simulink model "Model_pH_and_level_V1"  (Simulink 8.3)
settings: Solver=ode1  SolverMode=SingleTasking  StartTime=0.0  StopTime=Tsim  FixedStep=delta_sim  RelTol=1e-7
values from neighbouring files (symbols this model uses):
  b = 0    [Configuring_pH_and_level_model.m]
  delta_sim = 0.05    [Simulating_pH_and_level_model.m]
  e1 = 50    [Configuring_pH_and_level_model.m]
  e2 = 300    [Configuring_pH_and_level_model.m]
  filter_estimator1 = 1    [Configuring_pH_and_level_model.m]
  filter_estimator2 = 1    [Configuring_pH_and_level_model.m]
  filter_estimator3 = 1    [Configuring_pH_and_level_model.m]
  filter_estimator4 = 1    [Configuring_pH_and_level_model.m]
  filter_estimator5 = 1    [Configuring_pH_and_level_model.m]
  filter_estimator6 = 1    [Configuring_pH_and_level_model.m]
  filtro_Kp = fir1(5,1/50)    [Configuring_pH_and_level_model.m]
  filtro_med_F_TAPI = 1    [Configuring_pH_and_level_model.m]
  filtro_med_F_TASI = 1    [Configuring_pH_and_level_model.m]
  filtro_med_pH = 1    [Configuring_pH_and_level_model.m]
  filtro_Ti = fir1(5,1/50)    [Configuring_pH_and_level_model.m]
  h_max_TR_m = 0.5    [Configuring_pH_and_level_model.m]
  h_nom = 75    [Configuring_pH_and_level_model.m]
  I_l = 271.52    [Configuring_pH_and_level_model.m]
  K_meter_flow = 3600    [Configuring_pH_and_level_model.m]
  K_meter_level = 1    [Configuring_pH_and_level_model.m]
  K_meter_pH = 1    [Configuring_pH_and_level_model.m]
  Kc = 3.5    [Configuring_pH_and_level_model.m]
  Kn = 100/14    (= 7.14285714286)    [Configuring_pH_and_level_model.m]
  Kv = 11e-2    (= 0.11)    [Configuring_pH_and_level_model.m]
  mv0 = 50    [Configuring_pH_and_level_model.m]
  N = 1/500    (= 0.002)    [Configuring_pH_and_level_model.m]
  P_l = 11.65    [Configuring_pH_and_level_model.m]
  pH_nom = 7    [Configuring_pH_and_level_model.m]
  pka1_CH3COOH = interp1(Temp,pK_CH3COOH,T)    [Configuring_pH_and_level_model.m]
  pka1_H2CO3 = interp1(Temp,pK_H2CO3,T)    [Configuring_pH_and_level_model.m]
  pka1_H3PO4 = interp1(Temp,pK_H3PO4,T)    [Configuring_pH_and_level_model.m]
  pka1_NH4 = interp1(Temp,pK_NH4,T)    [Configuring_pH_and_level_model.m]
  pka2_H2CO3 = interp1(Temp,pK_HCO3,T)    [Configuring_pH_and_level_model.m]
  pka2_H3PO4 = interp1(Temp,pK_H2PO4,T)    [Configuring_pH_and_level_model.m]
  pka3_H3PO4 = interp1(Temp,pK_HPO4,T)    [Configuring_pH_and_level_model.m]
  pKw = interp1(Temp,pK_H2O,T)    [Configuring_pH_and_level_model.m]
  Q_ap_nom = 49/3600    (= 0.0136111111111)    [Configuring_pH_and_level_model.m]
  Qb_nom = c_HCl/c_NaOH*Q_ap_nom    (= 0.00412773748633)    [Configuring_pH_and_level_model.m]
  seed_noise_level = 12345    [Configuring_pH_and_level_model.m]
  seed_noise_pH = 67890    [Configuring_pH_and_level_model.m]
  seed_noise_Q_ap = 357    [Configuring_pH_and_level_model.m]
  seed_noise_Q_as = 349    [Configuring_pH_and_level_model.m]
  T_noise_level = 2    [Configuring_pH_and_level_model.m]
  T_noise_pH = 3    [Configuring_pH_and_level_model.m]
  T_PWM = 10    [Configuring_pH_and_level_model.m]
  tau_meter_flow = 1.4    [Configuring_pH_and_level_model.m]
  tau_meter_level = 16    [Configuring_pH_and_level_model.m]
  tau_meter_pH = 5    [Configuring_pH_and_level_model.m]
  Td = 120    [Configuring_pH_and_level_model.m]
  td_meter_flow = 3.5    [Configuring_pH_and_level_model.m]
  td_meter_level = 6    [Configuring_pH_and_level_model.m]
  td_meter_pH = 3.5    [Configuring_pH_and_level_model.m]
  Ti = 150    [Configuring_pH_and_level_model.m]
  Tmix = 1.34    [Configuring_pH_and_level_model.m]
  Ts = 0.5    [Simulating_pH_and_level_model.m]
  Ts_F_TAPI = 1    [Configuring_pH_and_level_model.m]
  Ts_F_TASI = 1    [Configuring_pH_and_level_model.m]
  Ts_Kp = 5    [Configuring_pH_and_level_model.m]
  Ts_pH_m = 1    [Configuring_pH_and_level_model.m]
  Ts_Ti = 5    [Configuring_pH_and_level_model.m]
  Ts_w1 = 1    [Configuring_pH_and_level_model.m]
  Ts_w2 = 1    [Configuring_pH_and_level_model.m]
  Ts_w3 = 1    [Configuring_pH_and_level_model.m]
  Ts_w4 = 1    [Configuring_pH_and_level_model.m]
  Ts_w5 = 1    [Configuring_pH_and_level_model.m]
  Ts_w6 = 25    [Configuring_pH_and_level_model.m]
  V0_CSTR = V_max_CSTR*h_nom/h_max_TR    (= 46.3491936722)    [Configuring_pH_and_level_model.m]
  V_max_CSTR = A_util_TR*h_max_TR_m*1000    (= 61.7989248962)    [Configuring_pH_and_level_model.m]
  var_noise_level = 1.1e-3    (= 0.0011)    [Configuring_pH_and_level_model.m]
  var_noise_pH = 6.25e-5    (= 6.25e-05)    [Configuring_pH_and_level_model.m]
  var_noise_Q_ap = 1.56e-2    (= 0.0156)    [Configuring_pH_and_level_model.m]
  var_noise_Q_as = 1.56e-2    (= 0.0156)    [Configuring_pH_and_level_model.m]
  Vm = 0.836    [Configuring_pH_and_level_model.m]
  w1_ff_tap = 0.0056    [Configuring_pH_and_level_model.m]
  w1_ff_tas = 0    [Configuring_pH_and_level_model.m]
  w1_ff_tbb = -0.0185    [Configuring_pH_and_level_model.m]
  w2_ff_tap = 0.5e-4    (= 5e-05)    [Configuring_pH_and_level_model.m]
  w2_ff_tbb = 0.5e-4    (= 5e-05)    [Configuring_pH_and_level_model.m]
  w3_ff_tap = 3e-4    (= 0.0003)    [Configuring_pH_and_level_model.m]
  w3_ff_tas = 3e-4    (= 0.0003)    [Configuring_pH_and_level_model.m]
  w3_ff_tbb = 3e-4    (= 0.0003)    [Configuring_pH_and_level_model.m]
  w4_ff_tap = 2e-4    (= 0.0002)    [Configuring_pH_and_level_model.m]
  w4_ff_tas = 2e-4    (= 0.0002)    [Configuring_pH_and_level_model.m]
  w4_ff_tbb = 2e-4    (= 0.0002)    [Configuring_pH_and_level_model.m]
  w_ap1 = c_HCl    (= 0.0055861204494)    [Configuring_pH_and_level_model.m]
  w_ap2 = c_CH3COOH_r    (= 0.0001)    [Configuring_pH_and_level_model.m]
  w_ap3 = c_H2CO3_r    (= 0.0009)    [Configuring_pH_and_level_model.m]
  w_ap4 = c_NH4    (= 0.0002)    [Configuring_pH_and_level_model.m]
  w_ap5 = c_H3PO4    (= 1e-05)    [Configuring_pH_and_level_model.m]
  w_as1 = 0    [Configuring_pH_and_level_model.m]
  w_as2 = c_CH3COOH    (= 0.00676612574825)    [Configuring_pH_and_level_model.m]
  w_as3 = c_H2CO3_r    (= 0.0009)    [Configuring_pH_and_level_model.m]
  w_as4 = c_NH4    (= 0.0002)    [Configuring_pH_and_level_model.m]
  w_as5 = c_H3PO4    (= 1e-05)    [Configuring_pH_and_level_model.m]
  w_b1 = -c_NaOH    (= -0.0184200924523)    [Configuring_pH_and_level_model.m]
  w_b2 = c_CH3COOH_r    (= 0.0001)    [Configuring_pH_and_level_model.m]
  w_b3 = c_H2CO3    (= 0.0005)    [Configuring_pH_and_level_model.m]
  w_b4 = c_NH4    (= 0.0002)    [Configuring_pH_and_level_model.m]
  w_b5 = c_H3PO4    (= 1e-05)    [Configuring_pH_and_level_model.m]
  w_fb_tap = [w1_ff_tap w2_ff_tap w3_ff_tap w4_ff_tap]    [Configuring_pH_and_level_model.m]
  w_fb_tas = [w1_ff_tas 0 w3_ff_tas w4_ff_tas]    [Configuring_pH_and_level_model.m]
  w_r1_0 = [w1_r1_0; c_CH3COOH_r; c_H2CO3_r; c_NH4; c_H3PO4]    [Configuring_pH_and_level_model.m]
  x_MV_pump = [0 10 20 40 50 60 80 100]    [Configuring_pH_and_level_model.m]
  y_Q_pump = Q_l_h/3600    [Configuring_pH_and_level_model.m]
libraries: simulink x6, simulink_extras x4
(part 1 of 2)
settings Model: Creator=BrIdent  LastModifiedBy=Fellipe
settings DataIOCC: Decimation=Decim  LimitDataPoints=off  SaveOutput=off  SignalLogging=off  TimeSaveName=t
settings OptimizationCC: ExpressionDepthLimit=2147483647
settings DebuggingCC: AlgebraicLoopMsg=none  ArtificialAlgebraicLoopMsg=none  SaveWithDisabledLinksMsg=none  SaveWithParameterizedLinksMsg=none  CheckSSInitialOutputMsg=off  MaxConsecutiveZCsMsg=none  SolverPrmCheckMsg=none  InheritedTsInSrcMsg=none  DiscreteInheritContinuousMsg=none  MultiTaskCondExecSysMsg=none  MultiTaskRateTransMsg=warning  TasksWithSamePriorityMsg=none  SigSpecEnsureSampleTimeMsg=none  Int32ToFloatConvMsg=none  ParameterDowncastMsg=none  ParameterOverflowMsg=none  InvalidFcnCallConnMsg=none  FcnCallInpInsideContextMsg=UseLocalSettings  UnconnectedInputMsg=none  UnconnectedOutputMsg=none  UnconnectedLineMsg=none  BusObjectLabelMismatch=none  RootOutportRequireBusObject=none  UnknownTsInhSupMsg=none  ModelReferenceDataLoggingMessage=none  ModelReferenceExtraNoncontSigs=none  StateNameClashWarn=none
settings ConfigurationSet: Description=SimMechanics 2G

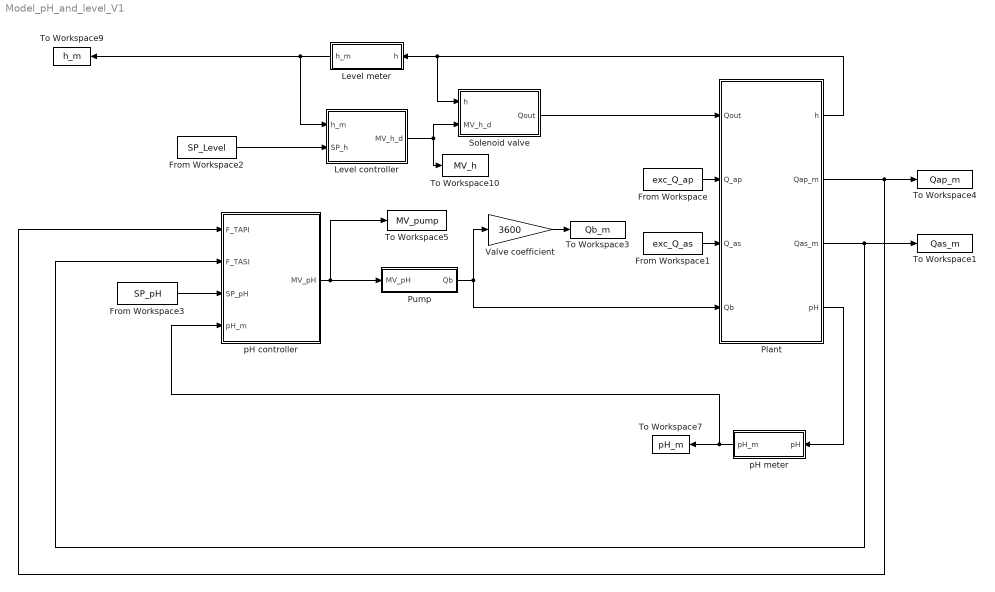
== system Model_pH_and_level_V1 ==
  From Workspace : FromWorkspace  VariableName=exc_Q_ap  SampleTime=1  Interpolate=off  OutputAfterFinalValue=Holding final value
  From Workspace1 : FromWorkspace  VariableName=exc_Q_as  SampleTime=1  Interpolate=off  OutputAfterFinalValue=Holding final value
  From Workspace2 : FromWorkspace  VariableName=SP_Level  SampleTime=1  Interpolate=off  OutputAfterFinalValue=Holding final value
  From Workspace3 : FromWorkspace  VariableName=SP_pH  SampleTime=1  Interpolate=off  OutputAfterFinalValue=Holding final value
  Level controller : Subsystem
  Level meter : Subsystem
  Plant : Subsystem
  Pump : Subsystem
  Solenoid valve : Subsystem
  To Workspace1 : ToWorkspace  VariableName=Qas_m  SampleTime=-1
      settings: Decimation=Ts/delta_sim
  To Workspace10 : ToWorkspace  VariableName=MV_h  SampleTime=-1
      settings: Decimation=Ts/delta_sim
  To Workspace3 : ToWorkspace  VariableName=Qb_m  SampleTime=-1
      settings: Decimation=Ts/delta_sim
  To Workspace4 : ToWorkspace  VariableName=Qap_m  SampleTime=-1
      settings: Decimation=Ts/delta_sim
  To Workspace5 : ToWorkspace  VariableName=MV_pump  SampleTime=-1
      settings: Decimation=Ts/delta_sim
  To Workspace7 : ToWorkspace  VariableName=pH_m  SampleTime=-1
      settings: Decimation=Ts/delta_sim
  To Workspace9 : ToWorkspace  VariableName=h_m  SampleTime=-1
      settings: Decimation=Ts/delta_sim
  Valve coefficient : Gain  Gain=3600
  pH controller : Subsystem  Description=Controlador
  pH meter : Subsystem
  wires:
  pH controller/1(MV_pH) -> To Workspace5/1, Pump/1(MV_pH)
  Plant/4(pH) -> pH meter/1(pH)
  Plant/1(h) -> Level meter/1(h), Solenoid valve/1(h)
  Pump/1(Qb) -> Valve coefficient/1, Plant/4(Qb)
  Plant/2(Qap_m) -> To Workspace4/1, pH controller/1(F_TAPI)
  From Workspace2/1 -> Level controller/2(SP_h)
  From Workspace3/1 -> pH controller/3(SP_pH)
  Level meter/1(h_m) -> Level controller/1(h_m), To Workspace9/1
  Solenoid valve/1(Qout) -> Plant/1(Qout)
  Level controller/1(MV_h_d) -> Solenoid valve/2(MV_h_d), To Workspace10/1
  From Workspace1/1 -> Plant/3(Q_as)
  Plant/3(Qas_m) -> To Workspace1/1, pH controller/2(F_TASI)
  From Workspace/1 -> Plant/2(Q_ap)
  Valve coefficient/1 -> To Workspace3/1
  pH meter/1(pH_m) -> pH controller/4(pH_m), To Workspace7/1

== system Model_pH_and_level_V1/Level controller ==
  h_m : Inport
  SP_h : Inport  Port=2
  PI Controller : simulink/Continuous/PID Controller  Controller=PI  TimeDomain=Discrete-time  SampleTime=Ts  IntegratorMethod=Trapezoidal  FilterMethod=Forward Euler  Form=Ideal  P=P_l  I=I_l  D=0  N=100  InitialConditionSource=internal  InitialConditionForIntegrator=0  InitialConditionForFilter=0  ExternalReset=none  LimitOutput=on  UpperSaturationLimit=100  LowerSaturationLimit=0  LinearizeAsGain=off  AntiWindupMode=back-calculation  Kb=1  TrackingMode=off  Kt=1  PParamMin=[]  PParamMax=[]  IParamMin=[]  IParamMax=[]  DParamMin=[]  DParamMax=[]  NParamMin=[]  NParamMax=[]  KbParamMin=[]  KbParamMax=[]  KtParamMin=[]  KtParamMax=[]  POutMin=[]  POutMax=[]  IOutMin=[]  IOutMax=[]  DOutMin=[]  DOutMax=[]  NOutMin=[]  NOutMax=[]  KbOutMin=[]  KbOutMax=[]  KtOutMin=[]  KtOutMax=[]  IntegratorOutMin=[]  IntegratorOutMax=[]  FilterOutMin=[]  FilterOutMax=[]  SumOutMin=[]  SumOutMax=[]  SumI1OutMin=[]  SumI1OutMax=[]  SumI2OutMin=[]  SumI2OutMax=[]  SumI3OutMin=[]  SumI3OutMax=[]  SumDOutMin=[]  SumDOutMax=[]  SaturationOutMin=[]  SaturationOutMax=[]  IntegratorContinuousStateAttributes=''  IntegratorStateMustResolveToSignalObject=off  IntegratorRTWStateStorageClass=Auto  FilterContinuousStateAttributes=''  FilterStateMustResolveToSignalObject=off  FilterRTWStateStorageClass=Auto
  PWM : Subsystem
  Sum : Sum  Inputs=-+
  MV_h_d : Outport
  wires:
  PI Controller/1 -> PWM/1(MV_h)
  PWM/1(MV_h_d) -> MV_h_d/1
  Sum/1 -> PI Controller/1  "e_h"
  h_m/1 -> Sum/2
  SP_h/1 -> Sum/1

== system Model_pH_and_level_V1/Level meter ==
  h : Inport
  1-D Lookup Table : Lookup_n-D  NumberOfTableDimensions=1  BreakpointsForDimension1=[53.78 62.05 70.32 83.51]  Table=[1.4 1.4 2.21 2.36]  ExtrapMethod=Clip  UseLastTableValue=on  InternalRulePriority=Speed  RndMeth=Simplest  InputSameDT=on
  Add : Sum
  Add1 : Sum
  Close : Constant  Value=0
  From Workspace : FromWorkspace  VariableName=mz81  Interpolate=off  OutputAfterFinalValue=Holding final value
  Level meter : simulink_extras/Additional Linear/Transfer Fcn (with initial outputs)  N=[K_meter_level]  D=[tau_meter_level 1]  Y0=h_nom  U0=h_nom
  Random Number : RandomNumber  Variance=var_noise_level  Seed=seed_noise_level  SampleTime=T_noise_level
  Switch : Switch  Criteria=u2 ~= 0
  Transport Delay : TransportDelay  DelayTime=td_meter_level  InitialOutput=h_nom
  h_m : Outport
  wires:
  h/1 -> 1-D Lookup Table/1, Level meter/1
  Level meter/1 -> Transport Delay/1
  Random Number/1 -> Add/2
  Transport Delay/1 -> Add/1
  Add/1 -> Add1/1
  Add1/1 -> h_m/1
  Close/1 -> Switch/3
  1-D Lookup Table/1 -> Switch/1
  From Workspace/1 -> Switch/2
  Switch/1 -> Add1/2

== system Model_pH_and_level_V1/Plant ==
  Qout : Inport
  Q_ap : Inport  Port=2
  Q_as : Inport  Port=3
  Qb : Inport  Port=4
  Flow meter Qap : Subsystem
  Flow meter Qas : Subsystem
  Plant : Subsystem
  h : Outport
  Qap_m : Outport  Port=2
  Qas_m : Outport  Port=3
  pH : Outport  Port=4
  wires:
  Plant/2(pH) -> pH/1
  Q_ap/1 -> Flow meter Qap/1(Qa), Plant/1(Q_ap)
  Qb/1 -> Plant/3(Qb)
  Flow meter Qap/1(Qap_m) -> Qap_m/1
  Q_as/1 -> Plant/2(Q_as), Flow meter Qas/1(Qa)
  Flow meter Qas/1(Qas_m) -> Qas_m/1
  Plant/1(h) -> h/1
  Qout/1 -> Plant/4(Qout)

== system Model_pH_and_level_V1/Pump ==
  MV_pH : Inport
  1-D Lookup Table : Lookup_n-D  NumberOfTableDimensions=1  BreakpointsForDimension1=x_MV_pump  Table=y_Q_pump  ExtrapMethod=Clip  RndMeth=Simplest  InputSameDT=on
  Qb : Outport
  wires:
  MV_pH/1 -> 1-D Lookup Table/1
  1-D Lookup Table/1 -> Qb/1

== system Model_pH_and_level_V1/Solenoid valve ==
  h : Inport
  MV_h_d : Inport  Port=2
  Conversion of level in % to meter : Gain  Gain=h_max_TR_m/100
  Product : Product  RndMeth=Zero
  Sqrt : Sqrt  SaturateOnIntegerOverflow=on
  Valve coefficient : Gain  Gain=Kv
  Qout : Outport
  wires:
  h/1 -> Conversion of level in % to meter/1
  Valve coefficient/1 -> Product/1
  MV_h_d/1 -> Valve coefficient/1
  Conversion of level in % to meter/1 -> Sqrt/1
  Sqrt/1 -> Product/2
  Product/1 -> Qout/1

== system Model_pH_and_level_V1/pH controller ==
  F_TAPI : Inport  Description=Qref
  F_TASI : Inport  Description=Qref  Port=2
  SP_pH : Inport  Description=Qref  Port=3
  pH_m : Inport  Description=Qref  Port=4
  Demux : Demux  Outputs=3
  Filter : Subsystem
  Mux : Mux  Inputs=3
  PID 2DOF + FF : Subsystem  Description=Controlador
  controller : Subsystem  Description=Controlador
  invariants estimator : Subsystem  Description=Controlador
  MV_pH : Outport
  wires:
  SP_pH/1 -> PID 2DOF + FF/1(SP_pH), controller/1(SP_pH)
  invariants estimator/1(w) -> controller/2(w)
  controller/1(MV_pH) -> MV_pH/1, invariants estimator/1(VM)
  F_TAPI/1 -> PID 2DOF + FF/3(Qap), invariants estimator/2(F_TAPI), Mux/1
  F_TASI/1 -> PID 2DOF + FF/4(Qas), invariants estimator/3(F_TASI), Mux/2
  pH_m/1 -> PID 2DOF + FF/2(pH_m), invariants estimator/4(pH_m), Mux/3
  Mux/1 -> Filter/1(U)
  Filter/1(Y) -> Demux/1
  Demux/1 -> controller/3(F_TAPI)
  Demux/2 -> controller/4(F_TASI)
  Demux/3 -> controller/5(pH_m)

== system Model_pH_and_level_V1/pH meter ==
  pH : Inport
  Add : Sum
  Random Number : RandomNumber  Variance=var_noise_pH  Seed=seed_noise_pH  SampleTime=T_noise_pH
  Transport Delay : TransportDelay  DelayTime=td_meter_pH  InitialOutput=pH_nom
  pH meter : simulink_extras/Additional Linear/Transfer Fcn (with initial outputs)  N=[K_meter_pH]  D=[tau_meter_pH 1]  Y0=pH_nom  U0=pH_nom
  pH_m : Outport
  wires:
  Transport Delay/1 -> Add/1
  Random Number/1 -> Add/2
  pH meter/1 -> Transport Delay/1
  pH/1 -> pH meter/1
  Add/1 -> pH_m/1

== system Model_pH_and_level_V1/Level controller/PWM ==
  MV_h : Inport
  Add1 : Sum  Inputs=++-
  Close : Constant  Value=0
  Compare to Zero : simulink/Logic and Bit Operations/Compare To Zero  relop=<=  OutDataTypeStr=boolean
  Constant : Constant  Value=50
  Open : Constant
  Sawtooth : SignalGenerator  WaveForm=sawtooth  Amplitude=50  Frequency=1/T_PWM
  Switch : Switch  Criteria=u2 > Threshold
  MV_h_d : Outport
  wires:
  Close/1 -> Switch/3
  Open/1 -> Switch/1
  Switch/1 -> MV_h_d/1
  Compare to Zero/1 -> Switch/2
  Constant/1 -> Add1/2
  MV_h/1 -> Add1/3
  Sawtooth/1 -> Add1/1
  Add1/1 -> Compare to Zero/1

== system Model_pH_and_level_V1/Plant/Flow meter Qap ==
  Qa : Inport
  Add : Sum
  Constant : Constant  Value=0
  Flow meter : simulink_extras/Additional Linear/Transfer Fcn (with initial outputs)  N=[K_meter_flow]  D=[tau_meter_flow 1]  Y0=0  U0=0
  Random Number : RandomNumber  Variance=var_noise_Q_ap  Seed=seed_noise_Q_ap  SampleTime=delta_sim
  Switch : Switch  Criteria=u2 > Threshold  Threshold=5/3600
  Transport Delay : TransportDelay  DelayTime=td_meter_flow
  Qap_m : Outport
  wires:
  Random Number/1 -> Add/2
  Qa/1 -> Switch/2, Flow meter/1
  Flow meter/1 -> Transport Delay/1
  Transport Delay/1 -> Add/1
  Add/1 -> Switch/1
  Constant/1 -> Switch/3
  Switch/1 -> Qap_m/1

== system Model_pH_and_level_V1/Plant/Flow meter Qas ==
  Qa : Inport
  Add : Sum
  Constant : Constant  Value=0
  Flow meter : simulink_extras/Additional Linear/Transfer Fcn (with initial outputs)  N=[K_meter_flow]  D=[tau_meter_flow 1]  Y0=0  U0=0
  Random Number : RandomNumber  Variance=var_noise_Q_as  Seed=seed_noise_Q_as  SampleTime=delta_sim
  Switch : Switch  Criteria=u2 > Threshold  Threshold=5/3600
  Transport Delay : TransportDelay  DelayTime=td_meter_flow
  Qas_m : Outport
  wires:
  Qa/1 -> Switch/2, Flow meter/1
  Random Number/1 -> Add/2
  Flow meter/1 -> Transport Delay/1
  Transport Delay/1 -> Add/1
  Constant/1 -> Switch/3
  Add/1 -> Switch/1
  Switch/1 -> Qas_m/1

== system Model_pH_and_level_V1/Plant/Plant ==
  Q_ap : Inport
  Q_as : Inport  Port=2
  Qb : Inport  Port=3
  Qout : Inport  Port=4
  Level model : Subsystem
  Simplified pH model : Subsystem  Description=Controlador
  pH model by reaction invariants : Subsystem
  h : Outport
  pH : Outport  Port=2
  wires:
  Level model/1(h) -> h/1
  pH model by reaction invariants/1(pH) -> pH/1
  Level model/2(V) -> pH model by reaction invariants/5(V)
  Q_ap/1 -> Simplified pH model/3(F_TASI), Level model/1(Q_ap), pH model by reaction invariants/1(Q_ap)
  Q_as/1 -> Simplified pH model/2(F_TAPI), Level model/2(Q_as), pH model by reaction invariants/2(Q_as)
  Qb/1 -> Simplified pH model/1(F_TBB), Level model/3(Qb), pH model by reaction invariants/3(Qb)
  Qout/1 -> Level model/4(Qout), pH model by reaction invariants/4(Qout)

== system Model_pH_and_level_V1/pH controller/Filter ==
  U : Inport
  Demux : Demux  Outputs=3
  Discrete FIR Filter : DiscreteFir  Coefficients=filtro_med_F_TAPI  SampleTime=Ts_F_TAPI
  Discrete FIR Filter1 : DiscreteFir  Coefficients=filtro_med_pH  InitialStates=pH_nom  SampleTime=Ts_pH_m
  Discrete FIR Filter2 : DiscreteFir  Coefficients=filtro_med_F_TASI  SampleTime=Ts_F_TASI
  Mux : Mux  Inputs=3
  Mux1 : Mux  Inputs=2
  Mux2 : Mux  Inputs=2
  Mux3 : Mux  Inputs=2
  Rate Transition3 : RateTransition  X0=pH_nom  OutPortSampleTime=Ts_pH_m
  Rate Transition4 : RateTransition  OutPortSampleTime=Ts_F_TASI
  Rate Transition5 : RateTransition  OutPortSampleTime=Ts_F_TAPI
  Rate Transition7 : RateTransition  X0=pH_nom
  Rate Transition8 : RateTransition
  Rate Transition9 : RateTransition
  Scope : Scope
      settings: YMax=15  SaveName=ScopeData12
  Scope1 : Scope
      settings: YMax=75  SaveName=ScopeData14
  Scope2 : Scope
      settings: YMin=4.4  YMax=6.5  SaveName=ScopeData15
  Y : Outport
  wires:
  U/1 -> Demux/1
  Mux/1 -> Y/1
  Demux/1 -> Rate Transition5/1, Mux1/2
  Rate Transition9/1 -> Mux1/1, Mux/1
  Mux1/1 -> Scope/1
  Demux/2 -> Rate Transition4/1, Mux2/2
  Mux2/1 -> Scope1/1
  Mux3/1 -> Scope2/1
  Discrete FIR Filter1/1 -> Rate Transition7/1
  Demux/3 -> Mux3/2, Rate Transition3/1
  Rate Transition3/1 -> Discrete FIR Filter1/1
  Rate Transition7/1 -> Mux/3, Mux3/1
  Rate Transition4/1 -> Discrete FIR Filter2/1
  Discrete FIR Filter2/1 -> Rate Transition8/1
  Rate Transition8/1 -> Mux2/1, Mux/2
  Rate Transition5/1 -> Discrete FIR Filter/1
  Discrete FIR Filter/1 -> Rate Transition9/1

== system Model_pH_and_level_V1/pH controller/PID 2DOF + FF ==
  note: e_pH
  note: e_pH
  SP_pH : Inport  Description=Qref
  pH_m : Inport  Description=Qref  Port=2
  Qap : Inport  Description=Qref  Port=3
  Qas : Inport  Description=Qref  Port=4
  Add : Sum  Inputs=+++
  Add1 : Sum  Inputs=|++-
  Add2 : Sum  Inputs=|+++
  Constant : Constant  Value=80
  Conversion from pH to %1 : Gain  Gain=Kn
  Conversion from pH to %2 : Gain  Gain=Kn
  Delay1 : Delay  DelayLength=1
  Delay2 : Delay  DelayLength=1
  Divide : Product  Inputs=*/
  Gain : Gain  Gain=0.8960
  PID Controller (2DOF) : simulink/Continuous/PID Controller (2DOF)  Controller=PID  TimeDomain=Discrete-time  SampleTime=1  IntegratorMethod=Forward Euler  FilterMethod=Forward Euler  Form=Ideal  P=Kc  I=1/Ti  D=Td  N=N  b=b  c=c  InitialConditionSource=internal  InitialConditionForIntegrator=50  InitialConditionForFilter=0  ExternalReset=none  LimitOutput=off  UpperSaturationLimit=inf  LowerSaturationLimit=-inf  LinearizeAsGain=on  AntiWindupMode=none  Kb=1  TrackingMode=off  Kt=1  PParamMin=[]  PParamMax=[]  IParamMin=[]  IParamMax=[]  DParamMin=[]  DParamMax=[]  NParamMin=[]  NParamMax=[]  bParamMin=[]  bParamMax=[]  cParamMin=[]  cParamMax=[]  KbParamMin=[]  KbParamMax=[]  KtParamMin=[]  KtParamMax=[]  POutMin=[]  POutMax=[]  IOutMin=[]  IOutMax=[]  DOutMin=[]  DOutMax=[]  NOutMin=[]  NOutMax=[]  bOutMin=[]  bOutMax=[]  cOutMin=[]  cOutMax=[]  KbOutMin=[]  KbOutMax=[]  KtOutMin=[]  KtOutMax=[]  IntegratorOutMin=[]  IntegratorOutMax=[]  FilterOutMin=[]  FilterOutMax=[]  SumOutMin=[]  SumOutMax=[]  Sum1OutMin=[]  Sum1OutMax=[]  Sum2OutMin=[]  Sum2OutMax=[]  Sum3OutMin=[]  Sum3OutMax=[]  SumI1OutMin=[]  SumI1OutMax=[]  SumI2OutMin=[]  SumI2OutMax=[]  SumI3OutMin=[]  SumI3OutMax=[]  SumDOutMin=[]  SumDOutMax=[]  SaturationOutMin=[]  SaturationOutMax=[]  IntegratorContinuousStateAttributes=''  IntegratorStateMustResolveToSignalObject=off  IntegratorRTWStateStorageClass=Auto  FilterContinuousStateAttributes=''  FilterStateMustResolveToSignalObject=off  FilterRTWStateStorageClass=Auto
  Transfer Fcn : TransferFcn  Numerator=[250 1]  Denominator=[241 1]
  x1 : Constant  Value=3
  x4 : Constant  Value=mv0
  MV_pH : Outport
  wires:
  x4/1 -> Add2/2
  Add2/1 -> MV_pH/1
  ? -> Add/3, Delay1/1
  Delay1/1 -> Add/2, Delay2/1
  Delay2/1 -> Add/1
  Add/1 -> Divide/1
  x1/1 -> Divide/2
  Gain/1 -> Transfer Fcn/1
  Qap/1 -> Add1/1
  Constant/1 -> Add1/3
  Qas/1 -> Add1/2
  Add1/1 -> Gain/1
  Transfer Fcn/1 -> Add2/3
  SP_pH/1 -> Conversion from pH to %2/1
  pH_m/1 -> Conversion from pH to %1/1
  Conversion from pH to %1/1 -> PID Controller (2DOF)/2
  PID Controller (2DOF)/1 -> Add2/1
  Conversion from pH to %2/1 -> PID Controller (2DOF)/1

== system Model_pH_and_level_V1/pH controller/controller ==
  note: FT(pHsp)
  note: û
  SP_pH : Inport  Description=Qref
  w : Inport  Description=Qref  Port=2
  F_TAPI : Inport  Description=Qref  Port=3
  F_TASI : Inport  Description=Qref  Port=4
  pH_m : Inport  Description=Qref  Port=5
  1-D Lookup Table : Lookup_n-D  NumberOfTableDimensions=1  BreakpointsForDimension1=y_Q_pump  Table=x_MV_pump  ExtrapMethod=Clip  RndMeth=Simplest  InputSameDT=on
  FB : Subsystem
  FF_1 : Subsystem
  FF_2 : Subsystem
  Gain4 : Gain  Gain=[0 0 0 0 0 1]  Multiplication=Matrix(K*u)
  Rate Transition : RateTransition  X0=50  OutPortSampleTime=Ts_F_TBB
  Rate Transition1 : RateTransition
  Scope : Scope
      settings: TimeRange=11000  YMin=-0.04  YMax=0.06  SaveName=ScopeData4
  Scope1 : Scope
      settings: YMin=0.00421  YMax=0.00438  SaveName=ScopeData5
  Scope2 : Scope
      settings: YMin=-0.0005  YMax=0.0075  SaveName=ScopeData9
  Sum5 : Sum  Inputs=+++
  MV_pH : Outport
  wires:
  w/1 -> Gain4/1, FB/3(w_TR)
  SP_pH/1 -> FF_2/1(SP_pH), FF_1/1(SP_pH), FB/2(SP_pH)
  F_TAPI/1 -> FB/4(F_TAPI), FF_1/2(F_TAPI)
  F_TASI/1 -> FB/5(F_TASI), FF_2/2(F_TASI)
  Gain4/1 -> [w2_TASI]
  Sum5/1 -> 1-D Lookup Table/1
  [w2_TASI] -> FF_2/3(w2_TASI)
  pH_m/1 -> FB/1(pH_m)
  FB/1(F_TBB) -> Sum5/1, Scope/1
  FF_1/1(F_TBB_1) -> Scope1/1, Sum5/2
  FF_2/1(F_TBB_2) -> Scope2/1, Sum5/3  "FT(pHsp)"
  Rate Transition/1 -> Rate Transition1/1
  1-D Lookup Table/1 -> Rate Transition/1
  Rate Transition1/1 -> MV_pH/1

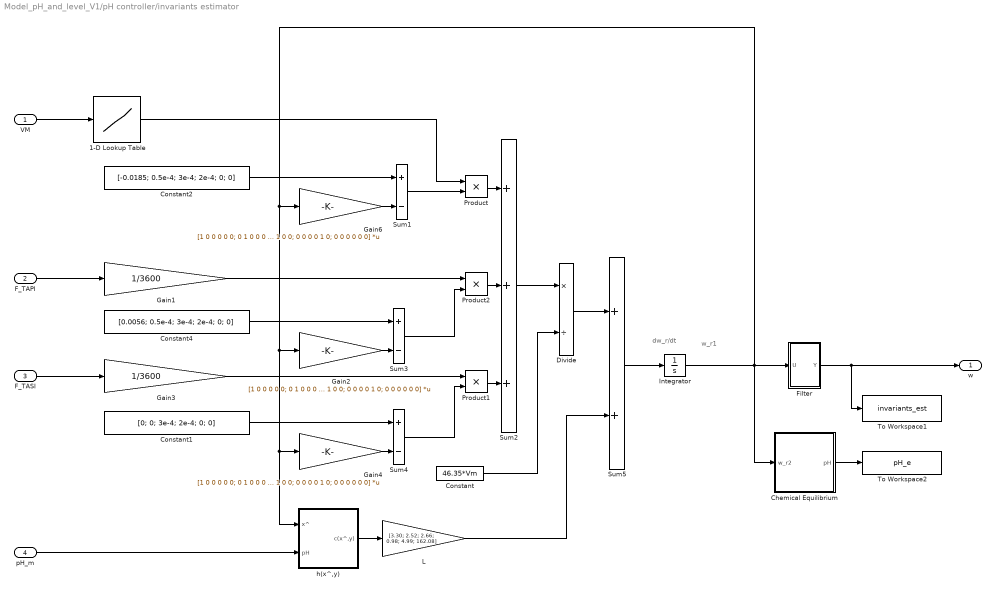
== system Model_pH_and_level_V1/pH controller/invariants estimator ==
  note: dw_r/dt
  note: w_r1
  VM : Inport  Description=Qref
  F_TAPI : Inport  Description=Qref  Port=2
  F_TASI : Inport  Description=Qref  Port=3
  pH_m : Inport  Description=Qref  Port=4
  1-D Lookup Table : Lookup_n-D  NumberOfTableDimensions=1  BreakpointsForDimension1=x_MV_pump  Table=y_Q_pump  ExtrapMethod=Clip  RndMeth=Simplest  InputSameDT=on
  Chemical Equilibrium : Subsystem
  Constant : Constant  Value=46.35*Vm
  Constant1 : Constant  Value=[0; 0; 3e-4; 2e-4; 0; 0]
  Constant2 : Constant  Value=[-0.0185; 0.5e-4; 3e-4; 2e-4; 0; 0]
  Constant4 : Constant  Value=[0.0056; 0.5e-4; 3e-4; 2e-4; 0; 0]
  Divide : Product  Inputs=*/
  Filter : Subsystem
  Gain1 : Gain  Gain=1/3600
  Gain2 : Gain  Gain=[1 0 0 0 0 0; 0 1 0 0 0 0; 0 0 1 0 0 0; 0 0 0 1 0 0; 0 0 0 0 1 0; 0 0 0 0 0 0]  Multiplication=Matrix(K*u)
  Gain3 : Gain  Gain=1/3600
  Gain4 : Gain  Gain=[1 0 0 0 0 0; 0 1 0 0 0 -1; 0 0 1 0 0 0; 0 0 0 1 0 0; 0 0 0 0 1 0; 0 0 0 0 0 0]  Multiplication=Matrix(K*u)
  Gain6 : Gain  Gain=[1 0 0 0 0 0; 0 1 0 0 0 0; 0 0 1 0 0 0; 0 0 0 1 0 0; 0 0 0 0 1 0; 0 0 0 0 0 0]  Multiplication=Matrix(K*u)
  Integrator : Integrator  InitialCondition=[0; 0; 0; 0; 0; 0]  LimitOutput=on  UpperSaturationLimit=[inf; inf; inf; inf; inf; inf]  LowerSaturationLimit=[-inf; 0; 0; 0; 0; 0]
  L : Gain  Gain=|
      | [3.30;
      | 2.52;
      | 2.66;
      | 0.98;
      | 4.99;
      | 162.08]
  Product : Product
  Product1 : Product
  Product2 : Product
  Sum1 : Sum  Inputs=+-
  Sum2 : Sum  Inputs=+++
  Sum3 : Sum  Inputs=+-
  Sum4 : Sum  Inputs=+-
  Sum5 : Sum
  To Workspace1 : ToWorkspace  VariableName=invariants_est  SampleTime=-1
      settings: Decimation=Ts/delta_sim
  To Workspace2 : ToWorkspace  VariableName=pH_e  SampleTime=-1
      settings: Decimation=Ts/delta_sim
  h(x^,y) : Subsystem
  w : Outport
  wires:
  Gain4/1 -> Sum4/2
  Gain3/1 -> Product1/1
  F_TASI/1 -> Gain3/1
  h(x^,y)/1(c(x^,y)) -> L/1
  Sum4/1 -> Product1/2
  Sum3/1 -> Product2/2
  Sum1/1 -> Product/2
  1-D Lookup Table/1 -> Product/1
  Constant2/1 -> Sum1/1
  Constant4/1 -> Sum3/1
  Constant1/1 -> Sum4/1
  Chemical Equilibrium/1(pH) -> To Workspace2/1
  Product1/1 -> Sum2/3
  Product/1 -> Sum2/1
  Product2/1 -> Sum2/2
  F_TAPI/1 -> Gain1/1
  VM/1 -> 1-D Lookup Table/1
  Gain1/1 -> Product2/1
  pH_m/1 -> h(x^,y)/2(pH)
  Integrator/1 -> Chemical Equilibrium/1(w_r2), Gain2/1, Gain4/1, h(x^,y)/1(x^), Gain6/1, Filter/1(U)
  Filter/1(Y) -> To Workspace1/1, w/1
  Sum5/1 -> Integrator/1
  Sum2/1 -> Divide/1
  Constant/1 -> Divide/2
  Divide/1 -> Sum5/1
  L/1 -> Sum5/2
  Gain2/1 -> Sum3/2
  Gain6/1 -> Sum1/2

== system Model_pH_and_level_V1/Plant/Plant/Level model ==
  Q_ap : Inport
  Q_as : Inport  Port=2
  Qb : Inport  Port=3
  Qout : Inport  Port=4
  A/H : Gain  Gain=100/V_max_CSTR
  Add : Sum  Inputs=+++-
  Integrator Limited : Integrator  InitialCondition=V0_CSTR  LimitOutput=on  UpperSaturationLimit=V_max_CSTR  LowerSaturationLimit=1e-6
  h : Outport
  V : Outport  Port=2
  wires:
  Q_ap/1 -> Add/1
  Add/1 -> Integrator Limited/1
  Integrator Limited/1 -> A/H/1, V/1
  A/H/1 -> h/1
  Qout/1 -> Add/4
  Qb/1 -> Add/3
  Q_as/1 -> Add/2

== system Model_pH_and_level_V1/Plant/Plant/Simplified pH model ==
  F_TBB : Inport  Description=Qref
  F_TAPI : Inport  Description=Qref  Port=2
  F_TASI : Inport  Description=Qref  Port=3
  Modelo da Planta Piloto : Subsystem
  wires:
  F_TBB/1 -> Modelo da Planta Piloto/1(F_TBB)
  F_TAPI/1 -> Modelo da Planta Piloto/2(F_TAPI)
  F_TASI/1 -> Modelo da Planta Piloto/3(F_TASI)

== system Model_pH_and_level_V1/Plant/Plant/pH model by reaction invariants ==
  note: w_r1
  note: dw_r/dt
  Q_ap : Inport
  Q_as : Inport  Port=2
  Qb : Inport  Port=3
  Qout : Inport  Port=4
  V : Inport  Port=5
  Add : Sum
  Add1 : Sum
  Chemical Equilibrium : Subsystem
  Constant1 : Constant  Value=[w_as1; w_as2; w_as3; w_as4; w_as5]
  Constant2 : Constant  Value=[w_ap1; w_ap2; w_ap3; w_ap4; w_ap5]
  Constant3 : Constant  Value=[w_b1; w_b2; w_b3; w_b4; w_b5]
  Constant8 : Constant  Value=0
  Divide : Product  Inputs=*/
  Gain2 : Gain  Gain=Vm
  Integrator : Integrator  InitialCondition=w_r1_0
  Product{,1..3} (4 alike) : Product
  Random Number : RandomNumber  Variance=[2e-10 0 0 0 0]  Seed=49863  SampleTime=delta_sim
  Random Number1 : RandomNumber  Variance=[0 1.5e-10 0 0 0]  Seed=4986947  SampleTime=delta_sim
  Scope : Scope
      settings: SaveName=ScopeData3
  Sum2 : Sum  Inputs=+++-
  To Workspace1 : ToWorkspace  VariableName=invariants  SampleTime=-1
      settings: Decimation=Ts/delta_sim
  Transport Delay : TransportDelay  DelayTime=Tmix  InitialOutput=Qb_nom
  Transport Delay1 : TransportDelay  DelayTime=Tmix
  Transport Delay2 : TransportDelay  DelayTime=Tmix  InitialOutput=Q_ap_nom
  ~=0 : Switch  Threshold=2/3600
  pH : Outport
  wires:
  Sum2/1 -> Divide/1
  V/1 -> Gain2/1
  Gain2/1 -> Divide/2
  Divide/1 -> Integrator/1
  Q_ap/1 -> Transport Delay2/1
  Qb/1 -> Transport Delay/1
  Product/1 -> Sum2/1
  Constant2/1 -> Product/1
  Q_as/1 -> Transport Delay1/1
  Constant1/1 -> Product2/1
  Product1/1 -> Sum2/3
  Integrator/1 -> Add/1, Product3/2
  Chemical Equilibrium/1(pH) -> pH/1
  Constant3/1 -> Product1/1
  Transport Delay1/1 -> ~=0/2, Product2/2
  Transport Delay2/1 -> Product/2
  Transport Delay/1 -> Product1/2
  Qout/1 -> Product3/1
  Product3/1 -> Sum2/4
  Random Number/1 -> Add/2
  Product2/1 -> Sum2/2
  Add/1 -> Add1/1
  ~=0/1 -> Add1/2
  Constant8/1 -> ~=0/3
  Random Number1/1 -> ~=0/1
  Add1/1 -> Chemical Equilibrium/1(w_r2), To Workspace1/1, Scope/1

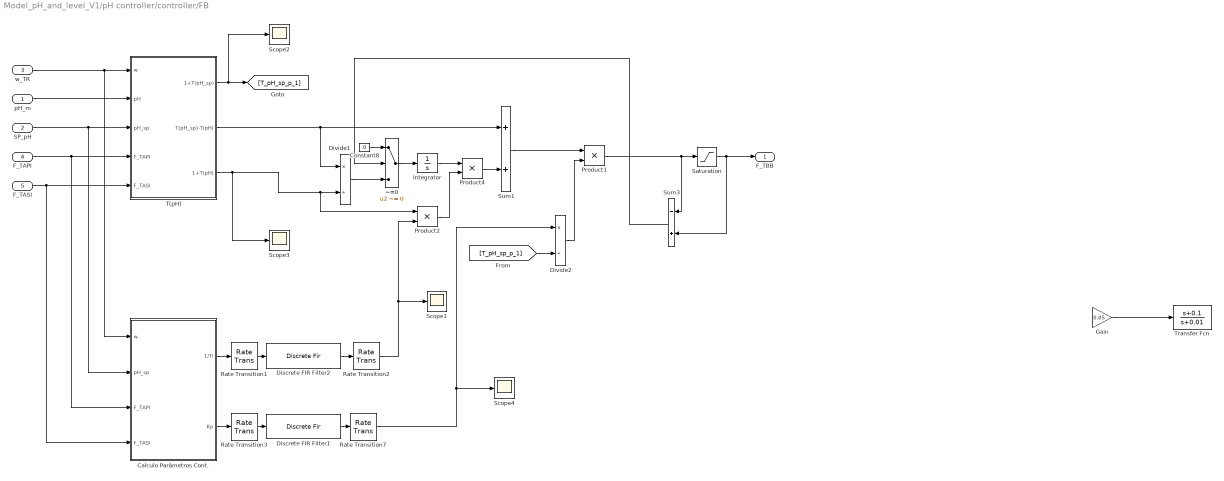
== system Model_pH_and_level_V1/pH controller/controller/FB ==
  pH_m : Inport  Description=Qref
  SP_pH : Inport  Description=Qref  Port=2
  w_TR : Inport  Description=Qref  Port=3
  F_TAPI : Inport  Description=Qref  Port=4
  F_TASI : Inport  Description=Qref  Port=5
  Calculo Parâmetros Cont. : Subsystem
  Constant8 : Constant  Value=0
  Discrete FIR Filter1 : DiscreteFir  Coefficients=filtro_Kp  SampleTime=Ts_Kp
  Discrete FIR Filter2 : DiscreteFir  Coefficients=filtro_Ti  SampleTime=Ts_Ti
  Divide1 : Product  Inputs=*/
  Divide2 : Product  Inputs=*/
  Gain : Gain  Gain=0.05
  Integrator : Integrator
  Product1 : Product
  Product2 : Product
  Product4 : Product
  Rate Transition1 : RateTransition  OutPortSampleTime=Ts_Ti
  Rate Transition2 : RateTransition
  Rate Transition3 : RateTransition  X0=pH_nom  OutPortSampleTime=Ts_Kp
  Rate Transition7 : RateTransition
  Saturation : Saturate  UpperLimit=10/3600  LowerLimit=-10/3600
  Scope{1..4} (4 alike) : Scope
      Scope1 settings: TimeRange=11000  YMin=0.0002  YMax=0.002  SaveName=ScopeData6
      Scope2 settings: TimeRange=11000  YMin=-0.75  YMax=2.5  SaveName=ScopeData7
      Scope3 settings: TimeRange=11000  YMin=-0.75  YMax=2.5  SaveName=ScopeData8
      Scope4 settings: TimeRange=11000  YMin=0.0002  YMax=0.002  SaveName=ScopeData11
  Sum1 : Sum
  Sum3 : Sum  Inputs=-+
  T(pH) : Subsystem
  Transfer Fcn : TransferFcn  Numerator=[1 0.1]  Denominator=[1 0.01]
  ~=0 : Switch  Criteria=u2 ~= 0
  F_TBB : Outport
  wires:
  Gain/1 -> Transfer Fcn/1
  w_TR/1 -> T(pH)/1(w), Calculo Parâmetros Cont./1(w)
  SP_pH/1 -> T(pH)/3(pH_sp), Calculo Parâmetros Cont./2(pH_sp)
  F_TAPI/1 -> T(pH)/4(F_TAPI), Calculo Parâmetros Cont./3(F_TAPI)
  F_TASI/1 -> T(pH)/5(F_TASI), Calculo Parâmetros Cont./4(F_TASI)
  Integrator/1 -> Product4/1
  Product4/1 -> Sum1/2
  Sum1/1 -> Product1/1
  Saturation/1 -> Sum3/2, F_TBB/1
  ~=0/1 -> Integrator/1
  Sum3/1 -> ~=0/2
  Constant8/1 -> ~=0/1
  Divide1/1 -> ~=0/3
  T(pH)/3(1+T(pH)) -> Scope3/1, Product2/1, Divide1/2
  Product2/1 -> Product4/2
  Divide2/1 -> Product1/2
  T(pH)/1(1+T(pH_sp)) -> Scope2/1, [T_pH_sp_p_1]
  [T_pH_sp_p_1] -> Divide2/2
  Product1/1 -> Sum3/1, Saturation/1
  Discrete FIR Filter1/1 -> Rate Transition7/1
  Rate Transition3/1 -> Discrete FIR Filter1/1
  Calculo Parâmetros Cont./2(Kp) -> Rate Transition3/1
  Rate Transition7/1 -> Scope4/1, Divide2/1
  Discrete FIR Filter2/1 -> Rate Transition2/1
  Rate Transition1/1 -> Discrete FIR Filter2/1
  Rate Transition2/1 -> Scope1/1, Product2/2
  Calculo Parâmetros Cont./1(1/Ti) -> Rate Transition1/1
  pH_m/1 -> T(pH)/2(pH)
  T(pH)/2(T(pH_sp)-T(pH)) -> Divide1/1, Sum1/1

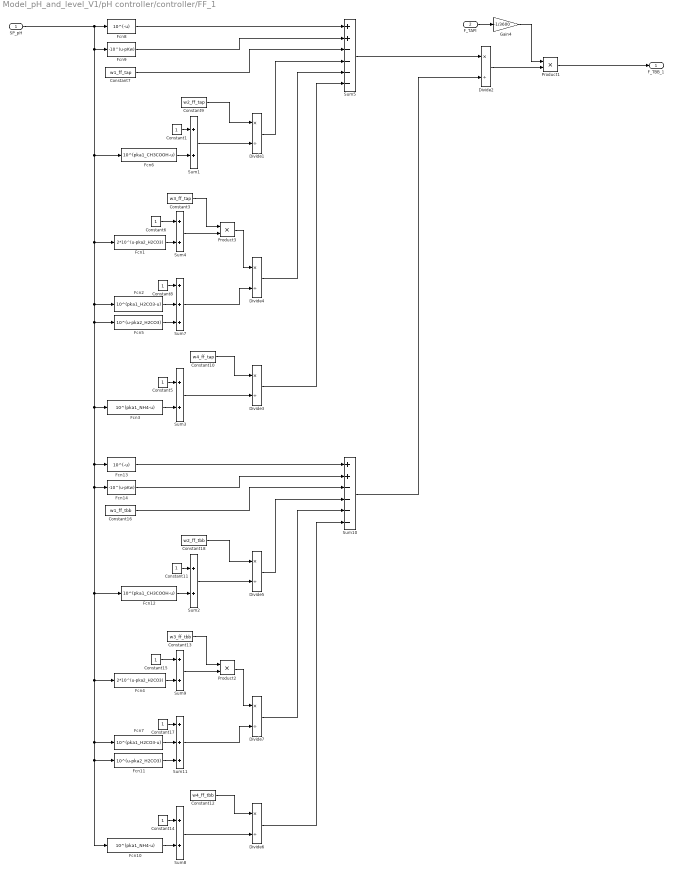
== system Model_pH_and_level_V1/pH controller/controller/FF_1 ==
  SP_pH : Inport  Description=Qref
  F_TAPI : Inport  Description=Qref  Port=2
  Constant{1,5..6,8,11,14..15,17} (8 alike) : Constant
  Constant10 : Constant  Value=w4_ff_tap
  Constant12 : Constant  Value=w4_ff_tbb
  Constant13 : Constant  Value=w3_ff_tbb
  Constant16 : Constant  Value=w1_ff_tbb
  Constant18 : Constant  Value=w2_ff_tbb
  Constant3 : Constant  Value=w3_ff_tap
  Constant7 : Constant  Value=w1_ff_tap
  Constant9 : Constant  Value=w2_ff_tap
  Divide{1..7} (7 alike) : Product  Inputs=*/
  Fcn1 : Fcn  Expr=2*10^(u-pka2_H2CO3)
  Fcn10 : Fcn  Expr=10^(pka1_NH4-u)
  Fcn11 : Fcn  Expr=10^(u-pka2_H2CO3)
  Fcn12 : Fcn  Expr=10^(pka1_CH3COOH-u)
  Fcn13 : Fcn  Expr=10^(-u)
  Fcn14 : Fcn  Expr=-10^(u-pKw)
  Fcn2 : Fcn  Expr=10^(pka1_H2CO3-u)
  Fcn3 : Fcn  Expr=10^(pka1_NH4-u)
  Fcn4 : Fcn  Expr=2*10^(u-pka2_H2CO3)
  Fcn5 : Fcn  Expr=10^(u-pka2_H2CO3)
  Fcn6 : Fcn  Expr=10^(pka1_CH3COOH-u)
  Fcn7 : Fcn  Expr=10^(pka1_H2CO3-u)
  Fcn8 : Fcn  Expr=10^(-u)
  Fcn9 : Fcn  Expr=-10^(u-pKw)
  Gain4 : Gain  Gain=-1/3600
  Product1 : Product
  Product2 : Product
  Product3 : Product
  Sum{1..4,8..9} (6 alike) : Sum
  Sum10 : Sum  Inputs=++----
  Sum11 : Sum  Inputs=+++
  Sum5 : Sum  Inputs=++----
  Sum7 : Sum  Inputs=+++
  F_TBB_1 : Outport
  wires:
  Sum4/1 -> Product3/2
  Product3/1 -> Divide4/1
  Constant6/1 -> Sum4/1
  Fcn5/1 -> Sum7/3
  Sum7/1 -> Divide4/2
  Fcn1/1 -> Sum4/2
  Fcn2/1 -> Sum7/2
  Constant8/1 -> Sum7/1
  Sum1/1 -> Divide1/2
  Fcn6/1 -> Sum1/2
  Constant1/1 -> Sum1/1
  Sum3/1 -> Divide3/2
  Fcn3/1 -> Sum3/2
  Constant5/1 -> Sum3/1
  Constant9/1 -> Divide1/1
  Constant3/1 -> Product3/1
  Constant10/1 -> Divide3/1
  Fcn8/1 -> Sum5/1
  Fcn9/1 -> Sum5/2
  Constant7/1 -> Sum5/3
  Divide1/1 -> Sum5/4
  Divide4/1 -> Sum5/5
  Divide3/1 -> Sum5/6
  Sum5/1 -> Divide2/1
  Divide2/1 -> Product1/2
  F_TAPI/1 -> Gain4/1
  Gain4/1 -> Product1/1
  Product1/1 -> F_TBB_1/1
  SP_pH/1 -> Fcn6/1, Fcn12/1, Fcn10/1, Fcn11/1, Fcn7/1, Fcn4/1, Fcn14/1, Fcn13/1, Fcn3/1, Fcn5/1, Fcn2/1, Fcn1/1, Fcn9/1, Fcn8/1
  Sum9/1 -> Product2/2
  Product2/1 -> Divide7/1
  Constant15/1 -> Sum9/1
  Fcn11/1 -> Sum11/3
  Sum11/1 -> Divide7/2
  Fcn4/1 -> Sum9/2
  Fcn7/1 -> Sum11/2
  Constant17/1 -> Sum11/1
  Sum2/1 -> Divide5/2
  Fcn12/1 -> Sum2/2
  Constant11/1 -> Sum2/1
  Sum8/1 -> Divide6/2
  Fcn10/1 -> Sum8/2
  Constant14/1 -> Sum8/1
  Constant18/1 -> Divide5/1
  Constant13/1 -> Product2/1
  Constant12/1 -> Divide6/1
  Fcn13/1 -> Sum10/1
  Fcn14/1 -> Sum10/2
  Constant16/1 -> Sum10/3
  Divide5/1 -> Sum10/4
  Divide7/1 -> Sum10/5
  Divide6/1 -> Sum10/6
  Sum10/1 -> Divide2/2

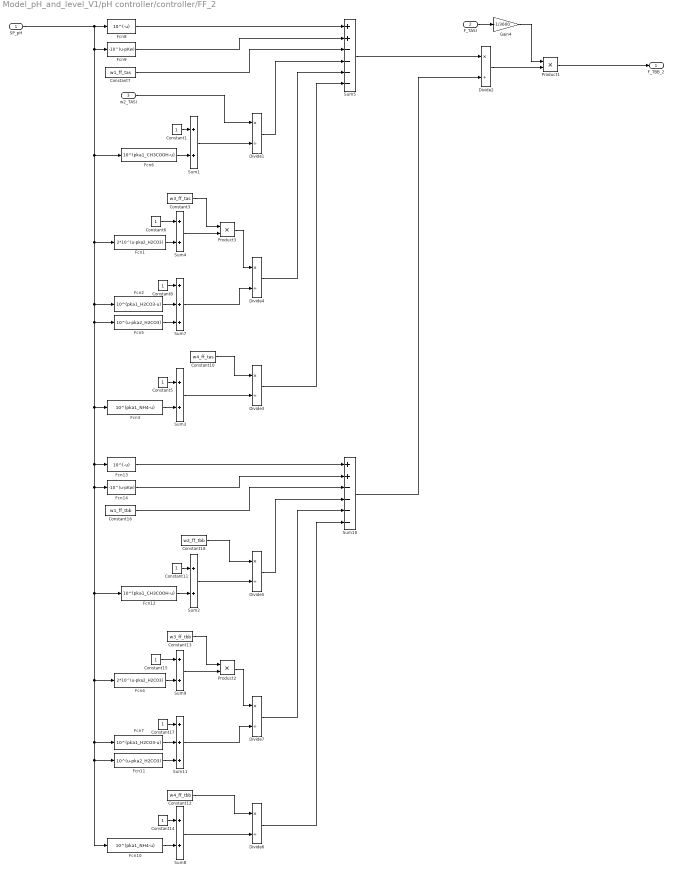
== system Model_pH_and_level_V1/pH controller/controller/FF_2 ==
  SP_pH : Inport  Description=Qref
  F_TASI : Inport  Description=Qref  Port=2
  w2_TASI : Inport  Description=Qref  Port=3
  Constant{1,5..6,8,11,14..15,17} (8 alike) : Constant
  Constant10 : Constant  Value=w4_ff_tas
  Constant12 : Constant  Value=w4_ff_tbb
  Constant13 : Constant  Value=w3_ff_tbb
  Constant16 : Constant  Value=w1_ff_tbb
  Constant18 : Constant  Value=w2_ff_tbb
  Constant3 : Constant  Value=w3_ff_tas
  Constant7 : Constant  Value=w1_ff_tas
  Divide{1..7} (7 alike) : Product  Inputs=*/
  Fcn1 : Fcn  Expr=2*10^(u-pka2_H2CO3)
  Fcn10 : Fcn  Expr=10^(pka1_NH4-u)
  Fcn11 : Fcn  Expr=10^(u-pka2_H2CO3)
  Fcn12 : Fcn  Expr=10^(pka1_CH3COOH-u)
  Fcn13 : Fcn  Expr=10^(-u)
  Fcn14 : Fcn  Expr=-10^(u-pKw)
  Fcn2 : Fcn  Expr=10^(pka1_H2CO3-u)
  Fcn3 : Fcn  Expr=10^(pka1_NH4-u)
  Fcn4 : Fcn  Expr=2*10^(u-pka2_H2CO3)
  Fcn5 : Fcn  Expr=10^(u-pka2_H2CO3)
  Fcn6 : Fcn  Expr=10^(pka1_CH3COOH-u)
  Fcn7 : Fcn  Expr=10^(pka1_H2CO3-u)
  Fcn8 : Fcn  Expr=10^(-u)
  Fcn9 : Fcn  Expr=-10^(u-pKw)
  Gain4 : Gain  Gain=-1/3600
  Product1 : Product
  Product2 : Product
  Product3 : Product
  Sum{1..4,8..9} (6 alike) : Sum
  Sum10 : Sum  Inputs=++----
  Sum11 : Sum  Inputs=+++
  Sum5 : Sum  Inputs=++----
  Sum7 : Sum  Inputs=+++
  F_TBB_2 : Outport
  wires:
  Sum10/1 -> Divide2/2
  Divide6/1 -> Sum10/6
  Divide7/1 -> Sum10/5
  Divide5/1 -> Sum10/4
  Constant16/1 -> Sum10/3
  Fcn14/1 -> Sum10/2
  Fcn13/1 -> Sum10/1
  Constant12/1 -> Divide6/1
  Constant13/1 -> Product2/1
  Constant18/1 -> Divide5/1
  Constant14/1 -> Sum8/1
  Fcn10/1 -> Sum8/2
  Sum8/1 -> Divide6/2
  Constant11/1 -> Sum2/1
  Fcn12/1 -> Sum2/2
  Sum2/1 -> Divide5/2
  Constant17/1 -> Sum11/1
  Fcn7/1 -> Sum11/2
  Fcn4/1 -> Sum9/2
  Sum11/1 -> Divide7/2
  Fcn11/1 -> Sum11/3
  Constant15/1 -> Sum9/1
  Product2/1 -> Divide7/1
  Sum9/1 -> Product2/2
  SP_pH/1 -> Fcn8/1, Fcn9/1, Fcn1/1, Fcn2/1, Fcn5/1, Fcn3/1, Fcn13/1, Fcn14/1, Fcn4/1, Fcn7/1, Fcn11/1, Fcn10/1, Fcn12/1, Fcn6/1
  Product1/1 -> F_TBB_2/1
  Gain4/1 -> Product1/1
  F_TASI/1 -> Gain4/1
  Divide2/1 -> Product1/2
  Sum5/1 -> Divide2/1
  Divide3/1 -> Sum5/6
  Divide4/1 -> Sum5/5
  Divide1/1 -> Sum5/4
  Constant7/1 -> Sum5/3
  Fcn9/1 -> Sum5/2
  Fcn8/1 -> Sum5/1
  Constant10/1 -> Divide3/1
  Constant3/1 -> Product3/1
  Constant5/1 -> Sum3/1
  Fcn3/1 -> Sum3/2
  Sum3/1 -> Divide3/2
  Constant1/1 -> Sum1/1
  Fcn6/1 -> Sum1/2
  Sum1/1 -> Divide1/2
  Constant8/1 -> Sum7/1
  Fcn2/1 -> Sum7/2
  Fcn1/1 -> Sum4/2
  Sum7/1 -> Divide4/2
  Fcn5/1 -> Sum7/3
  Constant6/1 -> Sum4/1
  Product3/1 -> Divide4/1
  Sum4/1 -> Product3/2
  w2_TASI/1 -> Divide1/1

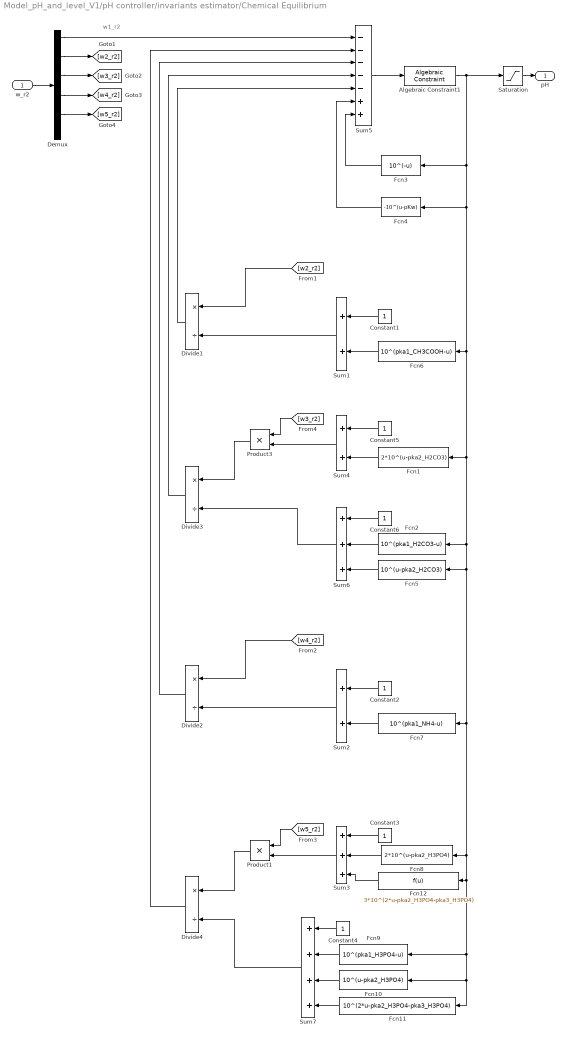
== system Model_pH_and_level_V1/pH controller/invariants estimator/Chemical Equilibrium ==
  note: w1_r2
  w_r2 : Inport
  Algebraic Constraint1 : simulink/Math Operations/Algebraic Constraint  z0=7
  Constant{1..6} (6 alike) : Constant
  Demux : Demux  Outputs=6
  Divide{1..4} (4 alike) : Product  Inputs=*/
  Fcn1 : Fcn  Expr=2*10^(u-pka2_H2CO3)
  Fcn10 : Fcn  Expr=10^(u-pka2_H3PO4)
  Fcn11 : Fcn  Expr=10^(2*u-pka2_H3PO4-pka3_H3PO4)
  Fcn12 : Fcn  Expr=3*10^(2*u-pka2_H3PO4-pka3_H3PO4)
  Fcn2 : Fcn  Expr=10^(pka1_H2CO3-u)
  Fcn3 : Fcn  Expr=10^(-u)
  Fcn4 : Fcn  Expr=-10^(u-pKw)
  Fcn5 : Fcn  Expr=10^(u-pka2_H2CO3)
  Fcn6 : Fcn  Expr=10^(pka1_CH3COOH-u)
  Fcn7 : Fcn  Expr=10^(pka1_NH4-u)
  Fcn8 : Fcn  Expr=2*10^(u-pka2_H3PO4)
  Fcn9 : Fcn  Expr=10^(pka1_H3PO4-u)
  Product1 : Product
  Product3 : Product
  Saturation : Saturate  UpperLimit=14  LowerLimit=0
  Sum1 : Sum
  Sum2 : Sum
  Sum3 : Sum  Inputs=+++
  Sum4 : Sum
  Sum5 : Sum  Inputs=-----++
  Sum6 : Sum  Inputs=+++
  Sum7 : Sum  Inputs=++++
  pH : Outport
  wires:
  Sum4/1 -> Product3/2
  Product3/1 -> Divide3/1
  Constant5/1 -> Sum4/1
  Algebraic Constraint1/1 -> Fcn3/1, Fcn6/1, Fcn1/1, Fcn2/1, Fcn5/1, Fcn12/1, Fcn9/1, Fcn10/1, Fcn11/1, Fcn8/1, Fcn7/1, Fcn4/1, Saturation/1
  Fcn5/1 -> Sum6/3
  Sum6/1 -> Divide3/2
  Sum5/1 -> Algebraic Constraint1/1
  Fcn1/1 -> Sum4/2
  Fcn2/1 -> Sum6/2
  Constant6/1 -> Sum6/1
  Saturation/1 -> pH/1
  w_r2/1 -> Demux/1
  Demux/1 -> Sum5/1
  Demux/2 -> [w2_r2]
  Demux/3 -> [w3_r2]
  [w3_r2] -> Product3/1
  [w2_r2] -> Divide1/1
  Sum1/1 -> Divide1/2
  Fcn6/1 -> Sum1/2
  Constant1/1 -> Sum1/1
  Demux/4 -> [w4_r2]
  [w4_r2] -> Divide2/1
  Sum2/1 -> Divide2/2
  Fcn7/1 -> Sum2/2
  Constant2/1 -> Sum2/1
  Fcn3/1 -> Sum5/7
  Fcn4/1 -> Sum5/6
  Sum3/1 -> Product1/2
  Product1/1 -> Divide4/1
  Constant3/1 -> Sum3/1
  Fcn10/1 -> Sum7/3
  Sum7/1 -> Divide4/2
  Fcn8/1 -> Sum3/2
  Fcn9/1 -> Sum7/2
  Constant4/1 -> Sum7/1
  [w5_r2] -> Product1/1
  Fcn11/1 -> Sum7/4
  Demux/5 -> [w5_r2]
  Divide1/1 -> Sum5/5
  Divide3/1 -> Sum5/4
  Divide2/1 -> Sum5/3
  Divide4/1 -> Sum5/2
  Fcn12/1 -> Sum3/3

== system Model_pH_and_level_V1/pH controller/invariants estimator/Filter ==
  U : Inport
  Demux : Demux  Outputs=6
  Discrete FIR Filter1 : DiscreteFir  Coefficients=filter_estimator1  SampleTime=Ts_w1
  Discrete FIR Filter2 : DiscreteFir  Coefficients=filter_estimator2  InitialStates=5e-5  SampleTime=Ts_w2
  Discrete FIR Filter3 : DiscreteFir  Coefficients=filter_estimator3  InitialStates=1e-4  SampleTime=Ts_w3
  Discrete FIR Filter4 : DiscreteFir  Coefficients=filter_estimator4  InitialStates=1e-4  SampleTime=Ts_w4
  Discrete FIR Filter5 : DiscreteFir  Coefficients=filter_estimator5  SampleTime=Ts_w5
  Discrete FIR Filter6 : DiscreteFir  Coefficients=filter_estimator6  SampleTime=Ts_w6
  Mux : Mux  Inputs=6
  Rate Transition : RateTransition  OutPortSampleTime=Ts_w5
  Rate Transition1 : RateTransition
  Rate Transition10 : RateTransition  OutPortSampleTime=Ts_w6
  Rate Transition11 : RateTransition
  Rate Transition2 : RateTransition  X0=1e-4  OutPortSampleTime=Ts_w4
  Rate Transition3 : RateTransition  X0=1e-4  OutPortSampleTime=Ts_w3
  Rate Transition4 : RateTransition  X0=5e-5  OutPortSampleTime=Ts_w2
  Rate Transition5 : RateTransition  OutPortSampleTime=Ts_w1
  Rate Transition6 : RateTransition  X0=1e-4
  Rate Transition7 : RateTransition  X0=1e-4
  Rate Transition8 : RateTransition  X0=5e-4
  Rate Transition9 : RateTransition
  Y : Outport
  wires:
  U/1 -> Demux/1
  Mux/1 -> Y/1
  Rate Transition8/1 -> Mux/2
  Rate Transition9/1 -> Mux/1
  Rate Transition1/1 -> Mux/5
  Rate Transition6/1 -> Mux/4
  Rate Transition7/1 -> Mux/3
  Demux/1 -> Rate Transition5/1
  Demux/2 -> Rate Transition4/1
  Demux/3 -> Rate Transition3/1
  Demux/4 -> Rate Transition2/1
  Demux/5 -> Rate Transition/1
  Rate Transition5/1 -> Discrete FIR Filter1/1
  Discrete FIR Filter1/1 -> Rate Transition9/1
  Rate Transition/1 -> Discrete FIR Filter5/1
  Discrete FIR Filter5/1 -> Rate Transition1/1
  Rate Transition2/1 -> Discrete FIR Filter4/1
  Rate Transition3/1 -> Discrete FIR Filter3/1
  Rate Transition4/1 -> Discrete FIR Filter2/1
  Discrete FIR Filter2/1 -> Rate Transition8/1
  Discrete FIR Filter3/1 -> Rate Transition7/1
  Discrete FIR Filter4/1 -> Rate Transition6/1
  Rate Transition10/1 -> Discrete FIR Filter6/1
  Discrete FIR Filter6/1 -> Rate Transition11/1
  Demux/6 -> Rate Transition10/1
  Rate Transition11/1 -> Mux/6

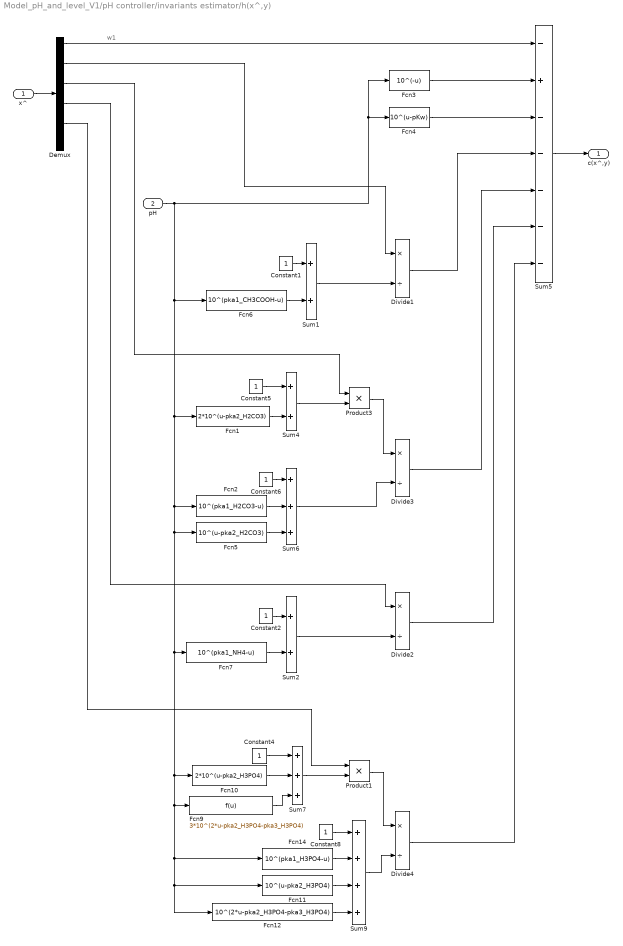
== system Model_pH_and_level_V1/pH controller/invariants estimator/h(x^,y) ==
  note: w1
  x^ : Inport
  pH : Inport  Port=2
  Constant{1..2,4..6,8} (6 alike) : Constant
  Demux : Demux  Outputs=6
  Divide{1..4} (4 alike) : Product  Inputs=*/
  Fcn1 : Fcn  Expr=2*10^(u-pka2_H2CO3)
  Fcn10 : Fcn  Expr=2*10^(u-pka2_H3PO4)
  Fcn11 : Fcn  Expr=10^(u-pka2_H3PO4)
  Fcn12 : Fcn  Expr=10^(2*u-pka2_H3PO4-pka3_H3PO4)
  Fcn14 : Fcn  Expr=10^(pka1_H3PO4-u)
  Fcn2 : Fcn  Expr=10^(pka1_H2CO3-u)
  Fcn3 : Fcn  Expr=10^(-u)
  Fcn4 : Fcn  Expr=10^(u-pKw)
  Fcn5 : Fcn  Expr=10^(u-pka2_H2CO3)
  Fcn6 : Fcn  Expr=10^(pka1_CH3COOH-u)
  Fcn7 : Fcn  Expr=10^(pka1_NH4-u)
  Fcn9 : Fcn  Expr=3*10^(2*u-pka2_H3PO4-pka3_H3PO4)
  Product1 : Product
  Product3 : Product
  Sum1 : Sum
  Sum2 : Sum
  Sum4 : Sum
  Sum5 : Sum  Inputs=-+-----
  Sum6 : Sum  Inputs=+++
  Sum7 : Sum  Inputs=+++
  Sum9 : Sum  Inputs=++++
  c(x^,y) : Outport
  wires:
  Divide2/1 -> Sum5/6
  Divide3/1 -> Sum5/5
  Divide1/1 -> Sum5/4
  Fcn4/1 -> Sum5/3
  Fcn3/1 -> Sum5/2
  Sum4/1 -> Product3/2
  Product3/1 -> Divide3/1
  Constant5/1 -> Sum4/1
  Fcn5/1 -> Sum6/3
  Sum6/1 -> Divide3/2
  Fcn1/1 -> Sum4/2
  Fcn2/1 -> Sum6/2
  Constant6/1 -> Sum6/1
  Sum5/1 -> c(x^,y)/1
  x^/1 -> Demux/1
  Demux/1 -> Sum5/1
  Demux/3 -> Product3/1
  Demux/2 -> Divide1/1
  Sum1/1 -> Divide1/2
  Fcn6/1 -> Sum1/2
  Constant1/1 -> Sum1/1
  Demux/4 -> Divide2/1
  Sum2/1 -> Divide2/2
  Fcn7/1 -> Sum2/2
  Constant2/1 -> Sum2/1
  pH/1 -> Fcn4/1, Fcn3/1, Fcn6/1, Fcn1/1, Fcn2/1, Fcn5/1, Fcn10/1, Fcn9/1, Fcn14/1, Fcn11/1, Fcn12/1, Fcn7/1
  Product1/1 -> Divide4/1
  Demux/5 -> Product1/1
  Fcn12/1 -> Sum9/4
  Fcn11/1 -> Sum9/3
  Fcn14/1 -> Sum9/2
  Constant8/1 -> Sum9/1
  Sum9/1 -> Divide4/2
  Constant4/1 -> Sum7/1
  Fcn10/1 -> Sum7/2
  Fcn9/1 -> Sum7/3
  Sum7/1 -> Product1/2
  Divide4/1 -> Sum5/7

== system Model_pH_and_level_V1/Plant/Plant/Simplified pH model/Modelo da Planta Piloto ==
  note: x^
  note: dx^/dt
  note: Ax^
  F_TBB : Inport  Description=Qref
  F_TAPI : Inport  Description=Qref  Port=2
  F_TASI : Inport  Description=Qref  Port=3
  Chemical Equilibrium : Subsystem
  Constant1 : Constant  Value=[-3.8955e-04 0 0 0 0; 0 -3.8955e-04 0 0 0; 0 0 -3.8955e-04 0 0; 0 0 0 -3.8955e-04 0; 0 0 0 0 -3.8955e-04]/Vm  VectorParams1D=off
  Constant2 : Constant  Value=[w_ap1 w_as1 w_b1; w_ap2 w_as2 w_b2; w_ap3 w_as3 w_b3; w_ap4 w_as4 w_b4; w_ap5 w_as5 w_b5]  VectorParams1D=off
  Constant3 : Constant  Value=15/3600
  Constant5 : Constant  Value=25/3600
  Constant6 : Constant  Value=25/3600
  Gain3 : Gain  Gain=1/46.35/Vm
  Gain4 : Gain  Gain=1/46.35/Vm
  Integrator : Integrator  InitialCondition=w_r1_0  LimitOutput=on  UpperSaturationLimit=[inf; inf; inf; inf; inf]  LowerSaturationLimit=[-inf; 0; 0; 0; 0]
  Mux : Mux  Inputs=3
  Product1 : Product  Inputs=**  Multiplication=Matrix(*)
  Product2 : Product
  Product3 : Product  Inputs=**  Multiplication=Matrix(*)
  Sum1 : Sum  Inputs=+-
  Sum3 : Sum  Inputs=+-
  Sum4 : Sum  Inputs=+-
  Sum5 : Sum  Inputs=+++
  Sum6 : Sum  Inputs=---
  To Workspace1 : ToWorkspace  VariableName=luenberger_est  SampleTime=-1
      settings: Decimation=Ts/delta_sim
  To Workspace2 : ToWorkspace  VariableName=pH_luen_e  SampleTime=-1
      settings: Decimation=Ts/delta_sim
  wires:
  Gain4/1 -> Sum5/3
  Product3/1 -> Gain4/1
  F_TBB/1 -> Sum1/1, Mux/3
  Mux/1 -> Product3/2
  Constant2/1 -> Product3/1
  Chemical Equilibrium/1(pH) -> To Workspace2/1
  Sum5/1 -> Integrator/1
  Product1/1 -> Sum5/2
  Constant1/1 -> Product1/1
  Gain3/1 -> Product2/2
  Sum6/1 -> Gain3/1
  Constant6/1 -> Sum4/2
  Constant5/1 -> Sum3/2
  Constant3/1 -> Sum1/2
  F_TAPI/1 -> Sum3/1, Mux/1
  F_TASI/1 -> Sum4/1, Mux/2
  Integrator/1 -> Chemical Equilibrium/1(w_r2), Product1/2, Product2/1, To Workspace1/1
  Sum3/1 -> Sum6/2
  Sum1/1 -> Sum6/3
  Sum4/1 -> Sum6/1
  Product2/1 -> Sum5/1

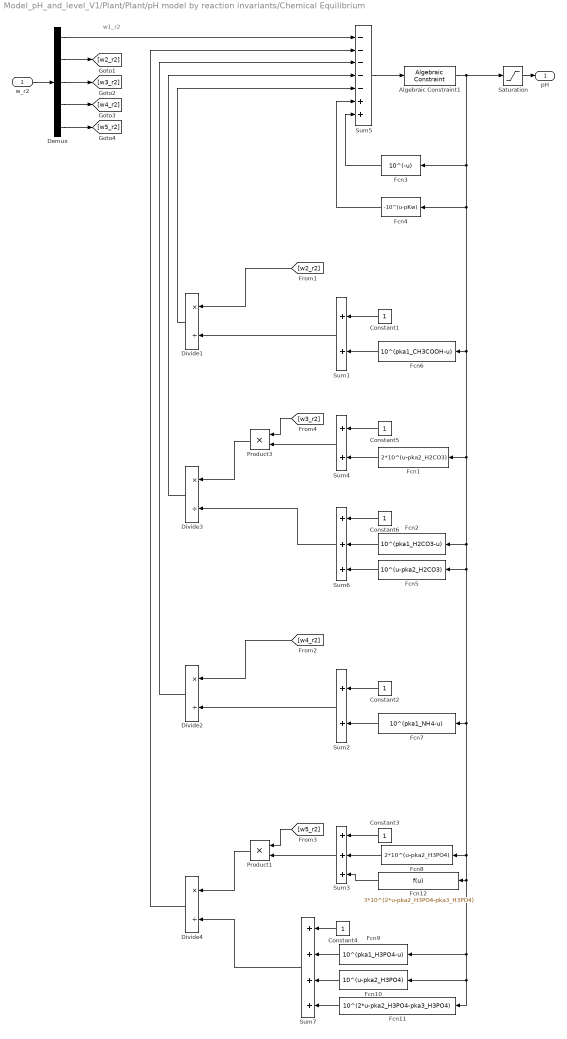
== system Model_pH_and_level_V1/Plant/Plant/pH model by reaction invariants/Chemical Equilibrium ==
  note: w1_r2
  w_r2 : Inport
  Algebraic Constraint1 : simulink/Math Operations/Algebraic Constraint  z0=7
  Constant{1..6} (6 alike) : Constant
  Demux : Demux  Outputs=5
  Divide{1..4} (4 alike) : Product  Inputs=*/
  Fcn1 : Fcn  Expr=2*10^(u-pka2_H2CO3)
  Fcn10 : Fcn  Expr=10^(u-pka2_H3PO4)
  Fcn11 : Fcn  Expr=10^(2*u-pka2_H3PO4-pka3_H3PO4)
  Fcn12 : Fcn  Expr=3*10^(2*u-pka2_H3PO4-pka3_H3PO4)
  Fcn2 : Fcn  Expr=10^(pka1_H2CO3-u)
  Fcn3 : Fcn  Expr=10^(-u)
  Fcn4 : Fcn  Expr=-10^(u-pKw)
  Fcn5 : Fcn  Expr=10^(u-pka2_H2CO3)
  Fcn6 : Fcn  Expr=10^(pka1_CH3COOH-u)
  Fcn7 : Fcn  Expr=10^(pka1_NH4-u)
  Fcn8 : Fcn  Expr=2*10^(u-pka2_H3PO4)
  Fcn9 : Fcn  Expr=10^(pka1_H3PO4-u)
  Product1 : Product
  Product3 : Product
  Saturation : Saturate  UpperLimit=14  LowerLimit=0
  Sum1 : Sum
  Sum2 : Sum
  Sum3 : Sum  Inputs=+++
  Sum4 : Sum
  Sum5 : Sum  Inputs=-----++
  Sum6 : Sum  Inputs=+++
  Sum7 : Sum  Inputs=++++
  pH : Outport
  wires:
  Sum4/1 -> Product3/2
  Product3/1 -> Divide3/1
  Constant5/1 -> Sum4/1
  Algebraic Constraint1/1 -> Fcn3/1, Fcn6/1, Fcn1/1, Fcn2/1, Fcn5/1, Fcn12/1, Fcn9/1, Fcn10/1, Fcn11/1, Fcn8/1, Fcn7/1, Fcn4/1, Saturation/1
  Fcn5/1 -> Sum6/3
  Sum6/1 -> Divide3/2
  Sum5/1 -> Algebraic Constraint1/1
  Fcn1/1 -> Sum4/2
  Fcn2/1 -> Sum6/2
  Constant6/1 -> Sum6/1
  Saturation/1 -> pH/1
  w_r2/1 -> Demux/1
  Demux/1 -> Sum5/1
  Demux/2 -> [w2_r2]
  Demux/3 -> [w3_r2]
  [w3_r2] -> Product3/1
  [w2_r2] -> Divide1/1
  Sum1/1 -> Divide1/2
  Fcn6/1 -> Sum1/2
  Constant1/1 -> Sum1/1
  Demux/4 -> [w4_r2]
  [w4_r2] -> Divide2/1
  Sum2/1 -> Divide2/2
  Fcn7/1 -> Sum2/2
  Constant2/1 -> Sum2/1
  Fcn3/1 -> Sum5/7
  Fcn4/1 -> Sum5/6
  Sum3/1 -> Product1/2
  Product1/1 -> Divide4/1
  Constant3/1 -> Sum3/1
  Fcn10/1 -> Sum7/3
  Sum7/1 -> Divide4/2
  Fcn8/1 -> Sum3/2
  Fcn9/1 -> Sum7/2
  Constant4/1 -> Sum7/1
  [w5_r2] -> Product1/1
  Fcn11/1 -> Sum7/4
  Demux/5 -> [w5_r2]
  Divide1/1 -> Sum5/5
  Divide3/1 -> Sum5/4
  Divide2/1 -> Sum5/3
  Divide4/1 -> Sum5/2
  Fcn12/1 -> Sum3/3
